simulink model "AGCProjectModel1copyCopy"  (R2020a)
settings: Solver=ode23t  StartTime=0.0  StopTime=100  RelTol=1e-3  AbsTol=1e-3  EnableMultiTasking=on
PreLoadFcn:
  | car_tire_data;
values from neighbouring files (symbols this model uses):
  rider_mass = 0    [car_tire_data.m]
  tire_dia = 18    [car_tire_data.m]
  vehicle_mass = 388    [car_tire_data.m]
libraries: fl_lib x18, nesl_utility x13, sdl_lib x6, ee_lib x2, fl_ps_legacy_lib x2, simulink x1
settings Model: Creator=sseshadr  LastModifiedBy=Ishmael
settings SolverCC: AutoScaleAbsTol=off
settings DataIOCC: LimitDataPoints=on  SaveFormat=Array  ReturnWorkspaceOutputs=off
settings OptimizationCC: LifeSpan=inf
settings DebuggingCC: SFUnexpectedBacktrackingDiag=warning  SFNoUnconditionalDefaultTransitionDiag=warning  SFExecutionAtInitializationDiag=none  ArithmeticOperatorsInVariantConditions=warning
settings HardwareCC: ProdBitPerPointer=32  ProdBitPerSizeT=32  ProdBitPerPtrDiffT=32  ProdLargestAtomicFloat=None  ProdIntDivRoundTo=Undefined  ProdEndianess=Unspecified  ProdWordSize=32  ProdHWDeviceType=32-bit Generic
settings ModelReferenceCC: PropagateSignalLabelsOutOfModel=off
settings SFSimCC: SimUseLocalCustomCode=off  CustomCodeUndefinedFunction=UseInterfaceOnly
settings RTWCC: RTWUseLocalCustomCode=off
settings CodeAppCC: StateflowObjectComments=on
settings GRTTargetCC: TargetLangStandard=C89/C90 (ANSI)
settings ConfigComp: CovMetricSettings=dw  CovHtmlReporting=on  CovSaveCumulativeToWorkspaceVar=on  CovSaveSingleToWorkspaceVar=on  CovExternalEMLEnable=off
settings SimscapeCC: SimscapeNormalizeSystem=off  SimscapeLogDataHistory=10000

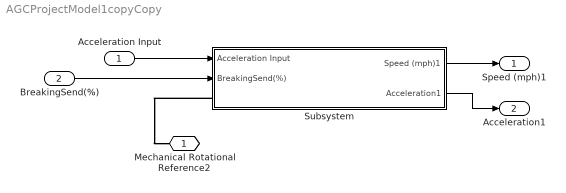
== system AGCProjectModel1copyCopy ==
  Acceleration Input : Inport
  BreakingSend(%) : Inport  Port=2
  Subsystem : Subsystem
  Mechanical Rotational Reference2 : PMIOPort  Side=Left
  Speed (mph)1 : Outport
  Acceleration1 : Outport  Port=2
  wires:
  Subsystem/1(Speed (mph)1) -> Speed (mph)1/1
  Subsystem/2(Acceleration1) -> Acceleration1/1
  Acceleration Input/1 -> Subsystem/1(Acceleration Input)
  BreakingSend(%)/1 -> Subsystem/2(BreakingSend(%))
  connections:
  Subsystem/LConn1 -- Mechanical Rotational Reference2/RConn1

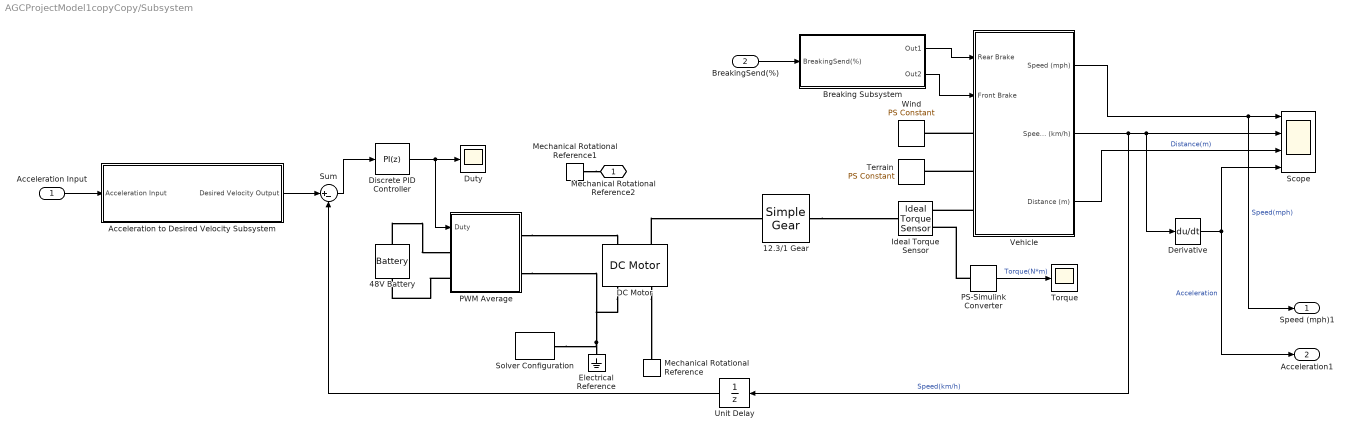
== system AGCProjectModel1copyCopy/Subsystem ==
  Acceleration Input : Inport
  BreakingSend(%) : Inport  Port=2
  12.3/1 Gear : sdl_lib/Gears/Simple Gear  ratio=12.3/1  rotation_direction=1  friction_model=sdl.enum.gear_efficiencies_load.off  T_noload=0.1 N*m  T_nom=5 N*m  efficiency_nom=0.8  efficiency=0.8  mu_visc=[ 0 0 ] N*m/(rad/s)  w_thr=0.01 rad/s  pwr_thr=0.001 W  enable_faults=simscape.enum.onoff.off  efficiency_fault=0.05  external_fault=simscape.enum.onoff.off  temporal_fault=simscape.enum.onoff.off  fault_time=5 s  fault_angles=pi / 12 rad  report_fault=1  temperature_TLU=[ 280 300 320 ] K  load_TLU=[ 1 5 10 ] N*m  efficiency_TLU=[ 0.95 0.9 0.85 ]  efficiency_TLU2=[ 0.85 0.8 0.75; 0.95 0.9 0.85; 0.85 0.8 0.7 ]  thermal_mass=50 J/K  T_init=300 K
  48V Battery : ee_lib/Sources/Battery  Vnom=48 V  R1=2 Ohm  prm_AH=1  AH=50 hr*A  V1=11.5 V  AH1=25 hr*A  prm_R2=1  R2=2000 Ohm  prm_dyn=1  Rp1=0.005 Ohm  tau1=30 s  Rp2=0.005 Ohm  tau2=30 s  Rp3=0.005 Ohm  tau3=30 s  Rp4=0.005 Ohm  tau4=30 s  Rp5=0.005 Ohm  tau5=30 s  prm_fade=1  N_fade=100  AH_fade=45 hr*A  R1_fade=2.02 Ohm  V1_fade=10.35 V  i_specify=off  i_priority=None  i=0 A  i_nominal_specify=off  i_nominal_unit=A  i_nominal_value=1  v_specify=off  v_priority=None  v=0 V  v_nominal_specify=off  v_nominal_unit=V  v_nominal_value=1  charge_specify=off  charge_priority=High  charge=50 hr*A  charge_nominal_specify=off  charge_nominal_unit=hr*A  charge_nominal_value=1  num_cycles_specify=off  num_cycles_priority=High  num_cycles=0  num_cycles_nominal_specify=off  num_cycles_nominal_unit=1  num_cycles_nominal_value=1  thermal_mass=30000 J/K  Tmeas=298.15 K  Vnom_T2=12 V  R1_T2=2.2 Ohm  V1_T2=11.4 V  R2_T2=2200 Ohm  Rp1_T2=0.005 Ohm  tau1_T2=30 s  Rp2_T2=0.005 Ohm  tau2_T2=30 s  Rp3_T2=0.005 Ohm  tau3_T2=30 s  Rp4_T2=0.005 Ohm  tau4_T2=30 s  Rp5_T2=0.005 Ohm  tau5_T2=30 s  Tmeas2=273.15 K  temperature_specify=off  temperature_priority=High  temperature=298.15 K  temperature_nominal_specify=off  temperature_nominal_unit=K  temperature_nominal_value=1
  Acceleration to Desired Velocity Subsystem : Subsystem
  Breaking Subsystem : Subsystem
  DC Motor : ee_lib/Electromechanical/Brushed Motors/DC Motor  field_option=ee.enum.field_option.pm  Rf=100 Ohm  Lf=1 H  Laf=0.15 H  If0=0 A  parameterization=1  Ra=0.0093 Ohm  La=172 uH  emf_or_torque=2  Kv=0.19 V/(rad/s)  Ki=0.19 N*m/A  T_stall=2.4e-4 N*m  w_max=1.91e+4 rpm  w_rated=1.5e+4 rpm  P_rated=0.08 W  V_rated=1.5 V  J=0.001 kg*m^2  lam_param=1  lam=1e-6 N*m/(rad/s)  i_noload=0 A  V_i_noload=1.5 V  speed0=0 rad/s  alpha=3.93e-3 1/K  Tmeas=25 degC  thermal_mass=100 J/K  initial_temperature=25 degC
  Derivative : Derivative
  Discrete PID Controller : simulink/Continuous/PID Controller  Controller=PI  Form=Parallel  TimeDomain=Discrete-time  UseExternalTs=off  SampleTime=0.05  IntegratorMethod=Forward Euler  FilterMethod=Forward Euler  ControllerParametersSource=internal  P=0.1  I=0.015  D=0  UseFilter=on  N=100  TunerSelectOption=Transfer Function Based (PID Tuner App)  InitialConditionSource=internal  InitialConditionForIntegrator=0  InitialConditionForFilter=0  DifferentiatorICPrevScaledInput=0  ExternalReset=none  TrackingMode=off  Kt=1  LimitOutput=on  UpperSaturationLimit=1  LowerSaturationLimit=0  LinearizeAsGain=off  AntiWindupMode=none  Kb=1  POutMin=[]  POutMax=[]  IOutMin=[]  IOutMax=[]  DOutMin=[]  DOutMax=[]  NOutMin=[]  NOutMax=[]  SumOutMin=[]  SumOutMax=[]  SaturationOutMin=[]  SaturationOutMax=[]  PParamMin=[]  PParamMax=[]  IParamMin=[]  IParamMax=[]  DParamMin=[]  DParamMax=[]  NParamMin=[]  NParamMax=[]  KbParamMin=[]  KbParamMax=[]  KtParamMin=[]  KtParamMax=[]  KbOutMin=[]  KbOutMax=[]  KtOutMin=[]  KtOutMax=[]  IntegratorOutMin=[]  IntegratorOutMax=[]  FilterOutMin=[]  FilterOutMax=[]  SumI1OutMin=[]  SumI1OutMax=[]  SumI2OutMin=[]  SumI2OutMax=[]  SumI3OutMin=[]  SumI3OutMax=[]  SumI4OutMin=[]  SumI4OutMax=[]  SumDOutMin=[]  SumDOutMax=[]  DifferentiatorOutMin=[]  DifferentiatorOutMax=[]  FilterDiffOutCoefMin=[]  FilterDiffOutCoefMax=[]  ReciprocalOutMin=[]  ReciprocalOutMax=[]  SumDenOutMin=[]  SumDenOutMax=[]  SumNumOutMin=[]  SumNumOutMax=[]  DivideOutMin=[]  DivideOutMax=[]  UdiffTsProdOutMin=[]  UdiffTsProdOutMax=[]  NTsProdOutMin=[]  NTsProdOutMax=[]  UintegralTsProdOutMin=[]  UintegralTsProdOutMax=[]  UngainTsProdOutMin=[]  UngainTsProdOutMax=[]  IntegratorContinuousStateAttributes=''  IntegratorStateMustResolveToSignalObject=off  IntegratorRTWStateStorageClass=Auto  FilterContinuousStateAttributes=''  FilterStateMustResolveToSignalObject=off  FilterRTWStateStorageClass=Auto  ParallelPVariant=InternalParameters  IdealPVariant=Disabled  IVariant=InternalParameters  DVariant=Disabled  IntegratorVariant=Discrete  SatVariant=Enabled  AWVariant=Passthrough  PCopyVariant=Disabled  TRVariant=Disabled  FdbkBlocksVariant=Forward  IdealPFdbkVariant=Disabled  SatFdbkVariant=Disabled  DerivativeFilterVariant=Disabled  NVariant=Disabled  NCopyVariant=Disabled_SignalSpec  FilterICVariant=Disabled  IntegratorICVariant=InternalICs  ExternalResetVariant=Disabled  TRSumVariant=Passthrough  SumFdbkVariant=Disabled  SumVariant=Sum_PI  TsampFilterVariant=InternalTs  TsampNgainVariant=Passthrough  TsampIntegralVariant=Passthrough
  Duty : Scope
  Electrical Reference : fl_lib/Electrical/Electrical Elements/Electrical Reference
  Ideal Torque Sensor : fl_lib/Mechanical/Mechanical Sensors/Ideal Torque Sensor
  Mechanical Rotational Reference : fl_lib/Mechanical/Rotational Elements/Mechanical Rotational Reference
  Mechanical Rotational Reference1 : fl_lib/Mechanical/Rotational Elements/Mechanical Rotational Reference
  PS-Simulink Converter : nesl_utility/PS-Simulink Converter  PhysicalDomain=network_engine_domain  SubClassName=ps_output  LeftPortType=input  RightPortType=output  PseudoPeriodic=off  Frequencies=[]  Unit=N*m  AffineConversion=off
  PWM Average : Subsystem
  Scope : Scope  NumInputPorts=4
  Solver Configuration : nesl_utility/Solver Configuration  PhysicalDomain=network_engine_domain  SubClassName=solver  LeftPortType=input  RightPortType=generic  Tones=[]  Harmonics=[]  SimulateNoise=off  Profile=off  UseLocalSampling=off  EnableSwitchedLinearOptims=on  FrequencyDomain=off  UseCCode=off  RelTol=0.001  AbsTol=1e-06  MinStep=1e-09  ToWorkspace=off  RevertToSquareIcSolve=off  NumHomotopyIterations=100  PhasorMode=off  PhasorModeNumHarmonics=1  DoDC=off  ResidualTolerance=1e-09  UseLocalSolver=off  LocalSolverChoice=NE_BACKWARD_EULER_ADVANCER  LocalSolverSampleTime=1e-7  DoFixedCost=off  MaxNonlinIter=3  MaxModeIter=2  LinearAlgebra=Sparse  EquationFormulation=NE_TIME_EF  DelaysMemoryBudget=1024  AutomaticFiltering=on  FilteringTimeConstant=0.001  PartitionStorageMethod=AS_NEEDED  PartitionMemoryBudget=1024  PartitionMethod=FAST
  Sum : Sum  Inputs=|+-
  Terrain : fl_lib/Physical Signals/Sources/PS Constant  constant=0
  Torque : Scope
  Unit Delay : UnitDelay  SampleTime=0.05  HasFrameUpgradeWarning=on
  Vehicle : Subsystem
  Wind : fl_lib/Physical Signals/Sources/PS Constant  constant=0
  Mechanical Rotational Reference2 : PMIOPort  Side=Left
  Speed (mph)1 : Outport
  Acceleration1 : Outport  Port=2
  wires:
  Vehicle/2(Speed (km/h)) -> Unit Delay/1, Derivative/1, Scope/2  "Speed(km/h)"
  Vehicle/3(Distance (m)) -> Scope/3  "Distance(m)"
  Derivative/1 -> Acceleration1/1, Scope/4  "Acceleration"
  Unit Delay/1 -> Sum/2
  Breaking Subsystem/1(Out1) -> Vehicle/1(Rear Brake)
  Vehicle/1(Speed (mph)) -> Speed (mph)1/1, Scope/1  "Speed(mph)"
  Sum/1 -> Discrete PID Controller/1
  Acceleration to Desired Velocity Subsystem/1(Desired Velocity Output) -> Sum/1
  BreakingSend(%)/1 -> Breaking Subsystem/1(BreakingSend(%))
  Acceleration Input/1 -> Acceleration to Desired Velocity Subsystem/1(Acceleration Input)
  Breaking Subsystem/2(Out2) -> Vehicle/2(Front Brake)
  PS-Simulink Converter/1 -> Torque/1  "Torque(N*m)"
  Discrete PID Controller/1 -> PWM Average/1(Duty), Duty/1
  connections:
  DC Motor/LConn2 -- 12.3/1 Gear/LConn1
  DC Motor/RConn2 -- Mechanical Rotational Reference/LConn1
  12.3/1 Gear/RConn1 -- Ideal Torque Sensor/LConn1
  PS-Simulink Converter/LConn1 -- Ideal Torque Sensor/RConn2
  48V Battery/LConn1 -- PWM Average/LConn1
  PWM Average/LConn2 -- 48V Battery/RConn1
  Electrical Reference/LConn1 -- Solver Configuration/RConn1 -- DC Motor/RConn1 -- PWM Average/RConn2
  Vehicle/LConn2 -- Terrain/RConn1
  Vehicle/LConn1 -- Wind/RConn1
  Vehicle/LConn3 -- Ideal Torque Sensor/RConn1
  Mechanical Rotational Reference1/LConn1 -- Mechanical Rotational Reference2/RConn1
  PWM Average/RConn1 -- DC Motor/LConn1

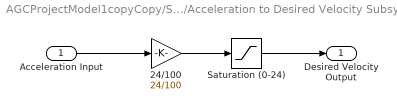
== system AGCProjectModel1copyCopy/Subsystem/Acceleration to Desired Velocity Subsystem ==
  Acceleration Input : Inport
  24/100 : Gain  Gain=24/100
  Saturation (0-24) : Saturate  UpperLimit=24  LowerLimit=0
  Desired Velocity Output : Outport
  wires:
  24/100/1 -> Saturation (0-24)/1
  Saturation (0-24)/1 -> Desired Velocity Output/1
  Acceleration Input/1 -> 24/100/1

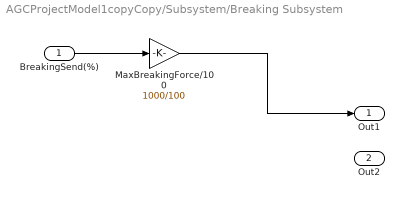
== system AGCProjectModel1copyCopy/Subsystem/Breaking Subsystem ==
  BreakingSend(%) : Inport
  MaxBreakingForce/100 : Gain  Gain=1000/100
  Out1 : Outport
  Out2 : Outport  Port=2
  wires:
  BreakingSend(%)/1 -> MaxBreakingForce/100/1
  MaxBreakingForce/100/1 -> Out1/1

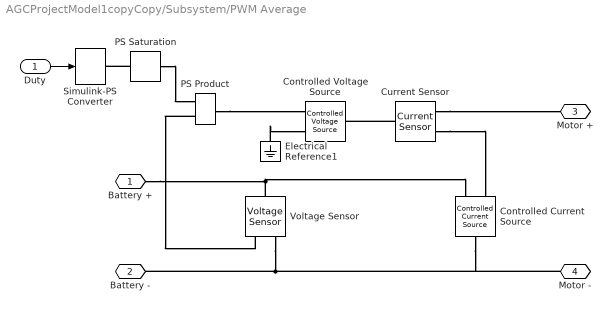
== system AGCProjectModel1copyCopy/Subsystem/PWM Average ==
  Duty : Inport
  Controlled Current Source : fl_lib/Electrical/Electrical Sources/Controlled Current Source
  Controlled Voltage Source : fl_lib/Electrical/Electrical Sources/Controlled Voltage Source
  Current Sensor : fl_lib/Electrical/Electrical Sensors/Current Sensor
  Electrical Reference1 : fl_lib/Electrical/Electrical Elements/Electrical Reference
  PS Product : fl_ps_legacy_lib/Legacy Physical Signals/Functions/PS Product
      settings: SourceProductBaseCode=SS
  PS Saturation : fl_ps_legacy_lib/Legacy Physical Signals/Nonlinear Operators/PS Saturation  upper_limit=1  lower_limit=0
      settings: SourceProductBaseCode=SS  InternalSimscapePortConfiguration="{\"Bottom\":[],\"Left\":[{\"id\":\"I\",\"label\":\"\",\"type\":\"input\"}],\"Right\":[{\"id\":\"O\",\"label\":\"\",\"type\":\"output\"}],\"Top\":[]}"
  Simulink-PS Converter : nesl_utility/Simulink-PS Converter  PhysicalDomain=network_engine_domain  SubClassName=ps_input  LeftPortType=input  RightPortType=output  PseudoPeriodic=off  Frequencies=[]  NoiseDistribution=none  NoiseParameters=[]  Unit=1  AffineConversion=off  FilteringAndDerivatives=zero  SimscapeFilterOrder=1  InputFilterTimeConstant=0.001  UdotUserProvided=1
  Voltage Sensor : fl_lib/Electrical/Electrical Sensors/Voltage Sensor
  Battery + : PMIOPort  Side=Left
  Battery - : PMIOPort  Port=2  Side=Left
  Motor + : PMIOPort  Port=3  Side=Right
  Motor - : PMIOPort  Port=4  Side=Right
  wires:
  Duty/1 -> Simulink-PS Converter/1
  connections:
  Electrical Reference1/LConn1 -- Controlled Voltage Source/RConn2
  Current Sensor/LConn1 -- Controlled Voltage Source/LConn1
  Voltage Sensor/RConn2 -- Controlled Current Source/LConn1 -- Motor -/RConn1 -- Battery -/RConn1
  Current Sensor/RConn1 -- Controlled Current Source/RConn1
  PS Product/LConn2 -- Voltage Sensor/RConn1
  Voltage Sensor/LConn1 -- Battery +/RConn1 -- Controlled Current Source/RConn2
  PS Product/RConn1 -- Controlled Voltage Source/RConn1
  Current Sensor/RConn2 -- Motor +/RConn1
  PS Saturation/RConn1 -- PS Product/LConn1
  PS Saturation/LConn1 -- Simulink-PS Converter/RConn1

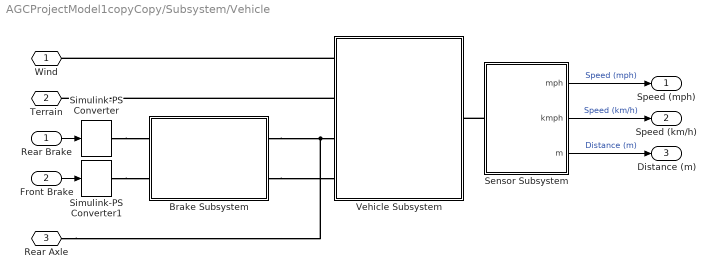
== system AGCProjectModel1copyCopy/Subsystem/Vehicle ==
  Rear Brake : Inport
  Front Brake : Inport  Port=2
  Brake Subsystem : Subsystem
  Sensor Subsystem : Subsystem
  Simulink-PS Converter : nesl_utility/Simulink-PS Converter  PhysicalDomain=network_engine_domain  SubClassName=ps_input  LeftPortType=input  RightPortType=output  PseudoPeriodic=off  Frequencies=[]  NoiseDistribution=none  NoiseParameters=[]  Unit=1  AffineConversion=off  FilteringAndDerivatives=filter  SimscapeFilterOrder=1  InputFilterTimeConstant=0.001  UdotUserProvided=1
  Simulink-PS Converter1 : nesl_utility/Simulink-PS Converter  PhysicalDomain=network_engine_domain  SubClassName=ps_input  LeftPortType=input  RightPortType=output  PseudoPeriodic=off  Frequencies=[]  NoiseDistribution=none  NoiseParameters=[]  Unit=1  AffineConversion=off  FilteringAndDerivatives=filter  SimscapeFilterOrder=1  InputFilterTimeConstant=0.001  UdotUserProvided=1
  Vehicle Subsystem : Subsystem
  Wind : PMIOPort  Side=Left
  Terrain : PMIOPort  Port=2  Side=Left
  Rear Axle : PMIOPort  Port=3  Side=Left
  Speed (mph) : Outport  VectorParamsAs1DForOutWhenUnconnected=off
  Speed (km/h) : Outport  Port=2  VectorParamsAs1DForOutWhenUnconnected=off
  Distance (m) : Outport  Port=3  VectorParamsAs1DForOutWhenUnconnected=off
  wires:
  Sensor Subsystem/1(mph) -> Speed (mph)/1  "Speed (mph)"
  Sensor Subsystem/2(kmph) -> Speed (km/h)/1  "Speed (km/h)"
  Sensor Subsystem/3(m) -> Distance (m)/1  "Distance (m)"
  Rear Brake/1 -> Simulink-PS Converter/1
  Front Brake/1 -> Simulink-PS Converter1/1
  connections:
  Simulink-PS Converter/RConn1 -- Brake Subsystem/LConn1
  Brake Subsystem/RConn1 -- Rear Axle/RConn1 -- Vehicle Subsystem/LConn3
  Brake Subsystem/RConn2 -- Vehicle Subsystem/LConn4
  Simulink-PS Converter1/RConn1 -- Brake Subsystem/LConn2
  Sensor Subsystem/LConn1 -- Vehicle Subsystem/RConn1
  Vehicle Subsystem/LConn1 -- Wind/RConn1
  Vehicle Subsystem/LConn2 -- Terrain/RConn1

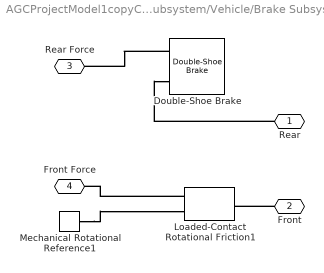
== system AGCProjectModel1copyCopy/Subsystem/Vehicle/Brake Subsystem ==
  Double-Shoe Brake : sdl_lib/Brakes & Detents/Rotational/Double-Shoe Brake  r_drum=150 mm  r_act=100 mm  r_pin=125 mm  theta_pin=15 deg  theta_0=5 deg  theta_shoe=120 deg  mu_visc=.01 N*m/(rad/s)  thermal_port=simscape.enum.thermaleffects.omit  mu=0.3  temperature_TLU=[280, 300, 320] K  mu_TLU=[.1, .05, .03]  thermal_mass=50 kJ/K  w_thr=0.01 rad/s  temperature_specify=off  temperature_priority=High  temperature=300 K  temperature_nominal_specify=off  temperature_nominal_unit=K  temperature_nominal_value=1
      settings: SourceProductBaseCode=LD  InternalSimscapePortConfiguration="{\"Bottom\":[],\"Left\":[{\"id\":\"F\",\"label\":\"F\",\"type\":\"input\"},{\"id\":\"S\",\"label\":\"S\",\"type\":\"foundation.mechanical.rotational.rotational\"}],\"Right\":[],\"Top\":[]}"
  Loaded-Contact Rotational Friction1 : sdl_lib/Brakes & Detents/Rotational/Loaded-Contact Rotational Friction  geometry_model=1  r_eff=280 mm  d_o=150 mm  d_i=100 mm  friction_model=1  mu_w_vector=[ 0 0.1 0.2 0.3 0.4 0.5 1 2 5 10 100 1000 ] rad/s  temperature_TLU=[280, 300, 320] K  mu_static=0.35  mu_static_vector=[.4, .38, .36]  mu_coulomb=0.3  mu_coulomb_vector=[ 0.29 0.28 0.26 0.22 0.21 0.2 0.2 0.19 0.19 0.19 0.19 0.19 ]  mu_coulomb_temp_vector=[.3, .28, .25]  mu_coulomb_matrix=[.34, .32, .3; .3, .28, .25; .25, .2, .15]  mu_interp_method=1  mu_extrap_method=1  w_tol=0.001 rad/s  force_min=1 N  mu_visc=0 N*m/(rad/s)  initial_state_locked=0  thermal_mass=50 kJ/K  T_init=300 K
      settings: SourceProductBaseCode=LD  InternalSimscapePortConfiguration="{\"Bottom\":[],\"Left\":[{\"id\":\"N\",\"label\":\"N\",\"type\":\"input\"},{\"id\":\"B\",\"label\":\"B\",\"type\":\"foundation.mechanical.rotational.rotational\"}],\"Right\":[{\"id\":\"F\",\"label\":\"F\",\"type\":\"foundation.mechanical.rotational.rotational\"}],\"Top\":[]}"
  Mechanical Rotational Reference1 : fl_lib/Mechanical/Rotational Elements/Mechanical Rotational Reference
  Rear : PMIOPort  Side=Right
  Front : PMIOPort  Port=2  Side=Right
  Rear Force : PMIOPort  Port=3  Side=Left
  Front Force : PMIOPort  Port=4  Side=Left
  connections:
  Mechanical Rotational Reference1/LConn1 -- Loaded-Contact Rotational Friction1/LConn2
  Double-Shoe Brake/LConn1 -- Rear Force/RConn1
  Loaded-Contact Rotational Friction1/LConn1 -- Front Force/RConn1
  Rear/RConn1 -- Double-Shoe Brake/LConn2
  Front/RConn1 -- Loaded-Contact Rotational Friction1/RConn1

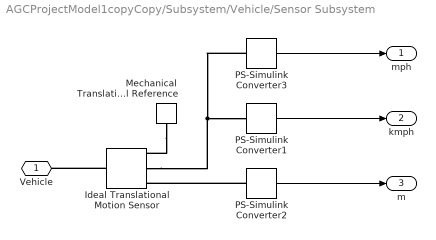
== system AGCProjectModel1copyCopy/Subsystem/Vehicle/Sensor Subsystem ==
  Ideal Translational Motion Sensor : fl_lib/Mechanical/Mechanical Sensors/Ideal Translational Motion Sensor  offset=0 m
  Mechanical Translational Reference : fl_lib/Mechanical/Translational Elements/Mechanical Translational Reference
  PS-Simulink Converter1 : nesl_utility/PS-Simulink Converter  PhysicalDomain=network_engine_domain  SubClassName=ps_output  LeftPortType=input  RightPortType=output  PseudoPeriodic=off  Frequencies=[]  Unit=km/hr  AffineConversion=off
  PS-Simulink Converter2 : nesl_utility/PS-Simulink Converter  PhysicalDomain=network_engine_domain  SubClassName=ps_output  LeftPortType=input  RightPortType=output  PseudoPeriodic=off  Frequencies=[]  Unit=1  AffineConversion=off
  PS-Simulink Converter3 : nesl_utility/PS-Simulink Converter  PhysicalDomain=network_engine_domain  SubClassName=ps_output  LeftPortType=input  RightPortType=output  PseudoPeriodic=off  Frequencies=[]  Unit=mph  AffineConversion=off
  Vehicle : PMIOPort  Side=Left
  mph : Outport  VectorParamsAs1DForOutWhenUnconnected=off
  kmph : Outport  Port=2  VectorParamsAs1DForOutWhenUnconnected=off
  m : Outport  Port=3  VectorParamsAs1DForOutWhenUnconnected=off
  wires:
  PS-Simulink Converter1/1 -> kmph/1
  PS-Simulink Converter2/1 -> m/1
  PS-Simulink Converter3/1 -> mph/1
  connections:
  Mechanical Translational Reference/LConn1 -- Ideal Translational Motion Sensor/RConn1
  PS-Simulink Converter2/LConn1 -- Ideal Translational Motion Sensor/RConn3
  Ideal Translational Motion Sensor/RConn2 -- PS-Simulink Converter3/LConn1 -- PS-Simulink Converter1/LConn1
  Ideal Translational Motion Sensor/LConn1 -- Vehicle/RConn1

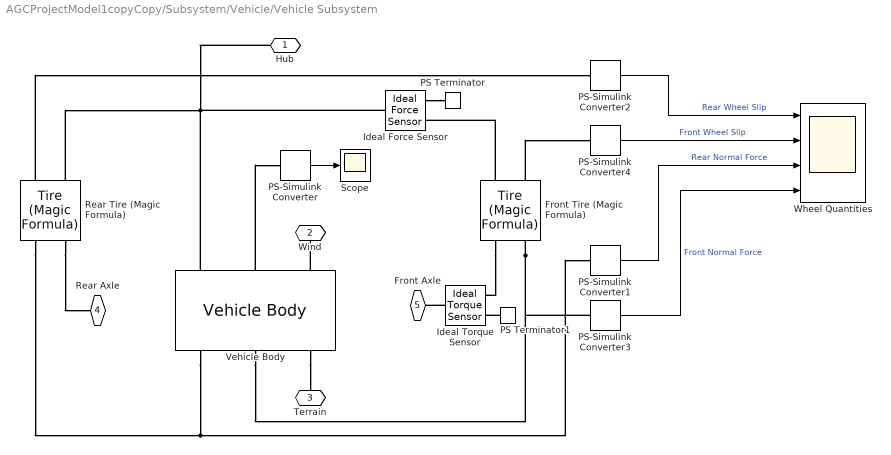
== system AGCProjectModel1copyCopy/Subsystem/Vehicle/Vehicle Subsystem ==
  Front Tire (Magic Formula) : sdl_lib/Tires & Vehicles/Tire (Magic Formula)  parameterization=sdl.enum.magic_tire_model.constant  F_z1=3e+3 N  F_x1=3.5e+3 N  kappa1=10  B_m=tire_b  C_m=tire_c  D_m=tire_d  E_m=tire_e  fz0=4e+3 N  p_Cx=1.685  p_Dx=[ 1.21 -0.037 ]  p_Ex=[ 0.344 0.095 -0.02 0 ]  p_Kx=[ 21.51 -0.163 0.245 ]  p_Hx=[ -0.002 0.002 ]  p_Vx=[ 0 0 ]  v_tr_thr=0.1 m/s  r_e=tire_dia/2 in  model_compliance=0  stiffness=1e+6 N/m  damping=1000 N/(m/s)  model_inertia=1  inertia=tire_inertia kg*m^2  initial_velocity=0 rad/s  model_resistance=1  resistance_model=1  coeff=roll_resist  p_tire=250e3 Pa  alpha=-0.003  beta=0.97  coeff_a=84e-4  coeff_b=6.2e-4 s/m  coeff_c=1.6e-4 s^2/m^2  v_thr=1e-3 m/s
  Ideal Force Sensor : fl_lib/Mechanical/Mechanical Sensors/Ideal Force Sensor
  Ideal Torque Sensor : fl_lib/Mechanical/Mechanical Sensors/Ideal Torque Sensor
  PS Terminator : fl_lib/Physical Signals/Sinks/PS Terminator
  PS Terminator1 : fl_lib/Physical Signals/Sinks/PS Terminator
  PS-Simulink Converter : nesl_utility/PS-Simulink Converter  PhysicalDomain=network_engine_domain  SubClassName=ps_output  LeftPortType=input  RightPortType=output  PseudoPeriodic=off  Frequencies=[]  Unit=1  AffineConversion=off
  PS-Simulink Converter{1..4} (4 alike) : nesl_utility/PS-Simulink Converter  PhysicalDomain=network_engine_domain  SubClassName=ps_output  LeftPortType=input  RightPortType=output  PseudoPeriodic=off  Frequencies=[]  Unit=N  AffineConversion=off
  Rear Tire (Magic Formula) : sdl_lib/Tires & Vehicles/Tire (Magic Formula)  parameterization=sdl.enum.magic_tire_model.constant  F_z1=3e+3 N  F_x1=3.5e+3 N  kappa1=10  B_m=tire_b  C_m=tire_c  D_m=tire_d  E_m=tire_e  fz0=4e+3 N  p_Cx=1.685  p_Dx=[ 1.21 -0.037 ]  p_Ex=[ 0.344 0.095 -0.02 0 ]  p_Kx=[ 21.51 -0.163 0.245 ]  p_Hx=[ -0.002 0.002 ]  p_Vx=[ 0 0 ]  v_tr_thr=0.1 m/s  r_e=tire_dia/2 in  model_compliance=0  stiffness=1e+6 N/m  damping=1000 N/(m/s)  model_inertia=1  inertia=tire_inertia kg*m^2  initial_velocity=0 rad/s  model_resistance=1  resistance_model=1  coeff=roll_resist  p_tire=250e3 Pa  alpha=-0.003  beta=0.97  coeff_a=84e-4  coeff_b=6.2e-4 s/m  coeff_c=1.6e-4 s^2/m^2  v_thr=1e-3 m/s
  Scope : Scope
  Vehicle Body : sdl_lib/Tires & Vehicles/Vehicle Body  mass=rider_mass + vehicle_mass kg  n_w=1  x_f=front_axle mm  x_r=rear_axle mm  y_c=CG_height mm  mass_var=simscape.enum.onoff.off  model_pitch=simscape.enum.onoff.off  inertia=4000 kg*m^2  suspension_model=sdl.enum.linearTLU.linear  k_f=1e4 N/m  b_f=1e4 N/(m/s)  k_r=1e4 N/m  b_r=1e4 N/(m/s)  k_f_TLU=[-2000, -1000, 0, 1000, 2000] N  x_f_TLU=[-.4, -.2, 0, .2, .4] m  b_f_TLU=[-200, -100, 0, 100, 200] N  v_f_TLU=[-4, -2, 0, 2, 4] m/s  k_r_TLU=[-2000, -1000, 0, 1000, 2000] N  x_r_TLU=[-.4, -.2, 0, .2, .4] m  b_r_TLU=[-200, -100, 0, 100, 200] N  v_r_TLU=[-4, -2, 0, 2, 4] m/s  interp_method=simscape.enum.interpolation.linear  extrap_method=simscape.enum.extrapolation.linear  model_hardstop=simscape.enum.onoff.off  upper_bound_f=.25 m  lower_bound_f=-.25 m  stop_k_f=1e6 N/m  stop_b_f=150 N/(m/s)  upper_bound_r=.25 m  lower_bound_r=-.25 m  stop_k_r=1e6 N/m  stop_b_r=150 N/(m/s)  initial_pitch=0 rad  initial_pitch_rate=0 rad/s  g=9.81 m/s^2  liftoff_warning=simscape.enum.onoff.off  area=front_area m^2  Cd=drag_coeff  rho=1.18 kg/m^3  v_specify=on  v_priority=High  v=0 m/s  v_nominal_specify=off  v_nominal_unit=m/s  v_nominal_value=1
  Wheel Quantities : Scope  NumInputPorts=4
  Hub : PMIOPort  Side=Right
  Wind : PMIOPort  Port=2  Side=Left
  Terrain : PMIOPort  Port=3  Side=Left
  Rear Axle : PMIOPort  Port=4  Side=Left
  Front Axle : PMIOPort  Port=5  Side=Left
  wires:
  PS-Simulink Converter/1 -> Scope/1
  PS-Simulink Converter2/1 -> Wheel Quantities/1  "Rear Wheel Slip"
  PS-Simulink Converter4/1 -> Wheel Quantities/2  "Front Wheel Slip"
  PS-Simulink Converter1/1 -> Wheel Quantities/3  "Rear Normal Force"
  PS-Simulink Converter3/1 -> Wheel Quantities/4  "Front Normal Force"
  connections:
  Vehicle Body/RConn1 -- Rear Tire (Magic Formula)/LConn1 -- PS-Simulink Converter1/LConn1
  Front Tire (Magic Formula)/LConn1 -- Vehicle Body/RConn2 -- PS-Simulink Converter3/LConn1
  Vehicle Body/LConn2 -- PS-Simulink Converter/LConn1
  Ideal Force Sensor/LConn1 -- Rear Tire (Magic Formula)/RConn2 -- Vehicle Body/LConn1 -- Hub/RConn1
  Vehicle Body/LConn3 -- Wind/RConn1
  Vehicle Body/RConn3 -- Terrain/RConn1
  Rear Tire (Magic Formula)/LConn2 -- Rear Axle/RConn1
  Front Tire (Magic Formula)/RConn2 -- Ideal Force Sensor/RConn1
  Ideal Torque Sensor/LConn1 -- Front Axle/RConn1
  Front Tire (Magic Formula)/LConn2 -- Ideal Torque Sensor/RConn1
  Front Tire (Magic Formula)/RConn1 -- PS-Simulink Converter4/LConn1
  Rear Tire (Magic Formula)/RConn1 -- PS-Simulink Converter2/LConn1
  Ideal Force Sensor/RConn2 -- PS Terminator/LConn1
  PS Terminator1/LConn1 -- Ideal Torque Sensor/RConn2
